simulink model "DC_Motor_Dynamic_Model"  (R2020a)
settings: Solver=VariableStepAuto  StartTime=0.0  StopTime=10.0  RelTol=1e-3
InitFcn:
  | Kf=.8;
  | TL=0;
  | 
  | Ra=.8;
  | La=5.8*10^(-3);
  | 
  | Rf=.2;
  | Lf=2*10^(-3);
  | 
  | Maf=0;
  | 
  | j=6.8*10^(-4);
  | B=.02;
settings Model: Creator=User  LastModifiedBy=User

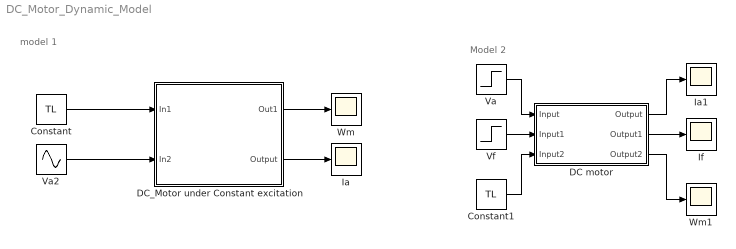
== system DC_Motor_Dynamic_Model ==
  note: Model 2
  note: model 1
  Constant : Constant  Value=TL
  Constant1 : Constant  Value=TL
  DC motor : Subsystem
  DC_Motor under Constant excitation : Subsystem
      mask Display:
      | image(imread('dcmotor.jpg'))
      | %color('red')
      | %port_label('input',1,'T_L')
      | %Port_label('input',2,'V_a')
      | 
      | %color('blue')
      | %port_label('output',1,'Wm')
      | %port_label('output',2,'I_a')
  Ia : Scope
  Ia1 : Scope
  If : Scope
  Va : Step  SampleTime=0
  Va2 : Sin  Amplitude=200  SampleTime=0
  Vf : Step  SampleTime=0
  Wm : Scope
  Wm1 : Scope
  wires:
  Constant/1 -> DC_Motor under Constant excitation/1(In1)
  Va2/1 -> DC_Motor under Constant excitation/2(In2)
  DC_Motor under Constant excitation/1(Out1) -> Wm/1
  DC_Motor under Constant excitation/2(Output) -> Ia/1
  Constant1/1 -> DC motor/3(Input2)
  Va/1 -> DC motor/1(Input)
  DC motor/3(Output2) -> Wm1/1
  DC motor/1(Output) -> Ia1/1
  DC motor/2(Output1) -> If/1
  Vf/1 -> DC motor/2(Input1)

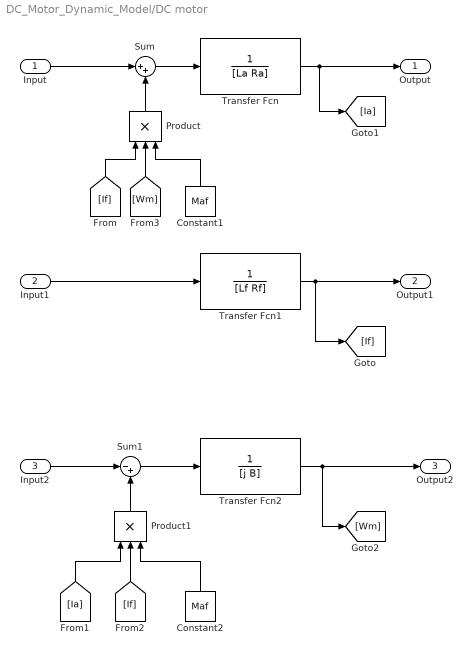
== system DC_Motor_Dynamic_Model/DC motor ==
  Input : Inport
  Input1 : Inport  Port=2
  Input2 : Inport  Port=3
  Constant1 : Constant  Value=Maf
  Constant2 : Constant  Value=Maf
  Product : Product  Inputs=3
  Product1 : Product  Inputs=3
  Sum : Sum  Inputs=|++
  Sum1 : Sum  Inputs=|-+
  Transfer Fcn : TransferFcn  Denominator=[La Ra]
  Transfer Fcn1 : TransferFcn  Denominator=[Lf Rf]
  Transfer Fcn2 : TransferFcn  Denominator=[j B]
  Output : Outport
  Output1 : Outport  Port=2
  Output2 : Outport  Port=3
  wires:
  Transfer Fcn/1 -> Output/1, [Ia]
  Product1/1 -> Sum1/2
  Input1/1 -> Transfer Fcn1/1
  Product/1 -> Sum/2
  Sum1/1 -> Transfer Fcn2/1
  Transfer Fcn1/1 -> Output1/1, [If]
  Transfer Fcn2/1 -> Output2/1, [Wm]
  Input/1 -> Sum/1
  Sum/1 -> Transfer Fcn/1
  [Ia] -> Product1/1
  [Wm] -> Product/2
  [If] -> Product1/2
  Input2/1 -> Sum1/1
  [If] -> Product/1
  Constant2/1 -> Product1/3
  Constant1/1 -> Product/3

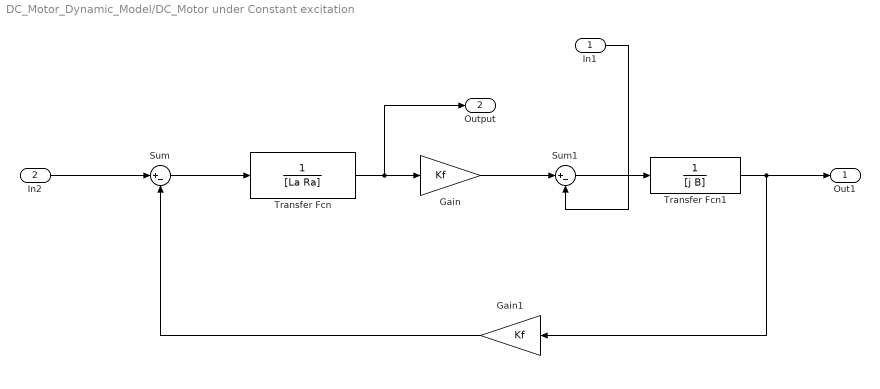
== system DC_Motor_Dynamic_Model/DC_Motor under Constant excitation ==
  In1 : Inport
  In2 : Inport  Port=2
  Gain : Gain  Gain=Kf
  Gain1 : Gain  Gain=Kf
  Sum : Sum  Inputs=|+-
  Sum1 : Sum  Inputs=|+-
  Transfer Fcn : TransferFcn  Denominator=[La Ra]
  Transfer Fcn1 : TransferFcn  Denominator=[j B]
  Out1 : Outport
  Output : Outport  Port=2
  wires:
  Sum/1 -> Transfer Fcn/1
  In2/1 -> Sum/1
  Transfer Fcn/1 -> Output/1, Gain/1
  Gain/1 -> Sum1/1
  Sum1/1 -> Transfer Fcn1/1
  Gain1/1 -> Sum/2
  Transfer Fcn1/1 -> Out1/1, Gain1/1
  In1/1 -> Sum1/2
